simulink subsystem "rss_ShuntMeasurementCircuit"  (R2022b)
settings: Solver=VariableStepAuto  StartTime=0.0  StopTime=10.0  RelTol=1e-3
undefined symbols (not defined in the file): cstShntFiltRstn, cstShntRstn
libraries: fl_lib x10, nesl_utility x1
settings Model: Creator=CAV2OFO  LastModifiedBy=CAV2OFO

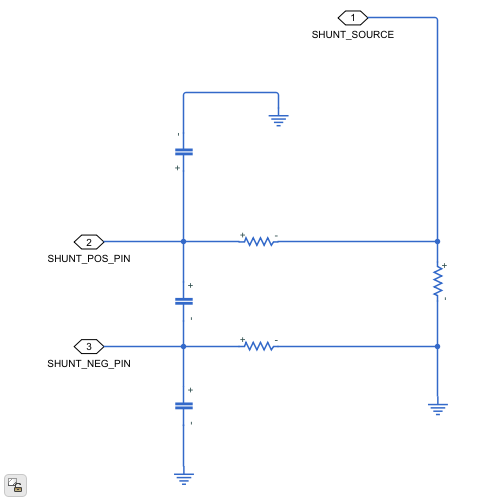
[thumbnail: Simulink's stored preview of the top-level diagram]
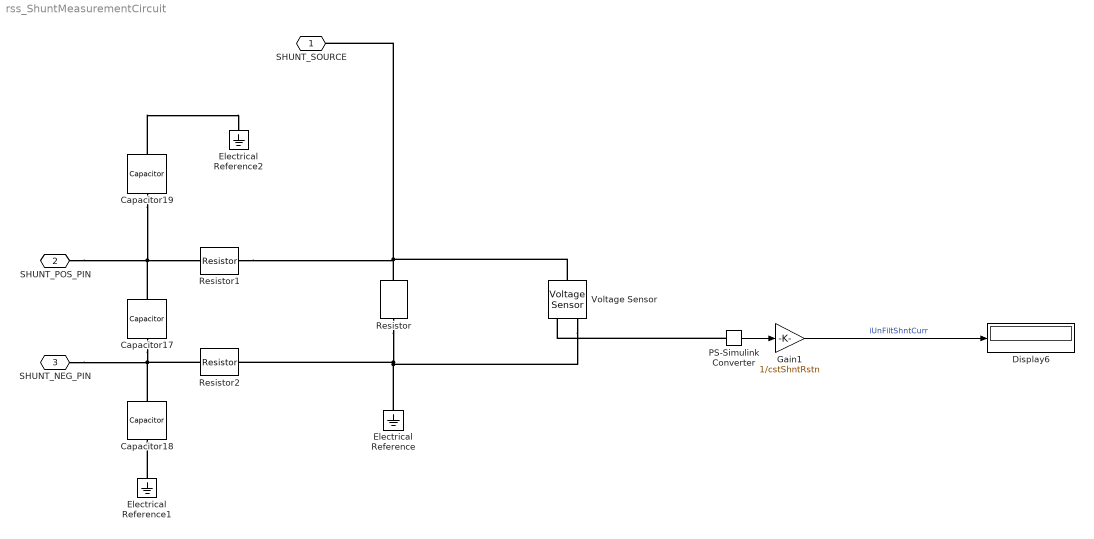
== system rss_ShuntMeasurementCircuit ==
  Capacitor17 : fl_lib/Electrical/Electrical Elements/Capacitor  c=cstShntCpct F  r=cstShntCpcrRstn Ohm  g=0 1/Ohm  i_specify=off  i_priority=None  i=0 A  i_nominal_specify=off  i_nominal_unit=A  i_nominal_value=1  v_specify=off  v_priority=None  v=0 V  v_nominal_specify=off  v_nominal_unit=V  v_nominal_value=1  vc_specify=off  vc_priority=High  vc=0 V  vc_nominal_specify=off  vc_nominal_unit=V  vc_nominal_value=1
  Capacitor18 : fl_lib/Electrical/Electrical Elements/Capacitor  c=cstShntGrndCpct F  r=cstShntGrndCpcrRstn Ohm  g=0 1/Ohm  i_specify=off  i_priority=None  i=0 A  i_nominal_specify=off  i_nominal_unit=A  i_nominal_value=1  v_specify=off  v_priority=None  v=0 V  v_nominal_specify=off  v_nominal_unit=V  v_nominal_value=1  vc_specify=off  vc_priority=High  vc=0 V  vc_nominal_specify=off  vc_nominal_unit=V  vc_nominal_value=1
  Capacitor19 : fl_lib/Electrical/Electrical Elements/Capacitor  c=cstShntGrndCpct F  r=cstShntGrndCpcrRstn Ohm  g=0 1/Ohm  i_specify=off  i_priority=None  i=0 A  i_nominal_specify=off  i_nominal_unit=A  i_nominal_value=1  v_specify=off  v_priority=None  v=0 V  v_nominal_specify=off  v_nominal_unit=V  v_nominal_value=1  vc_specify=off  vc_priority=High  vc=0 V  vc_nominal_specify=off  vc_nominal_unit=V  vc_nominal_value=1
  Display6 : Display
  Electrical Reference : fl_lib/Electrical/Electrical Elements/Electrical Reference
  Electrical Reference1 : fl_lib/Electrical/Electrical Elements/Electrical Reference
  Electrical Reference2 : fl_lib/Electrical/Electrical Elements/Electrical Reference
  Gain1 : Gain  Gain=1/cstShntRstn
  PS-Simulink Converter : nesl_utility/PS-Simulink Converter  PhysicalDomain=network_engine_domain  SubClassName=ps_output  LeftPortType=input  RightPortType=output  PseudoPeriodic=off  Frequencies=[]  VectorFormat=inherit  Unit=inherit  AffineConversion=off
  Resistor : fl_lib/Electrical/Electrical Elements/Resistor  R=cstShntRstn Ohm  i_specify=off  i_priority=None  i=0 A  i_nominal_specify=off  i_nominal_unit=A  i_nominal_value=1  v_specify=off  v_priority=None  v=0 V  v_nominal_specify=off  v_nominal_unit=V  v_nominal_value=1
  Resistor1 : fl_lib/Electrical/Electrical Elements/Resistor  R=cstShntFiltRstn Ohm  i_specify=off  i_priority=None  i=0 A  i_nominal_specify=off  i_nominal_unit=A  i_nominal_value=1  v_specify=off  v_priority=None  v=0 V  v_nominal_specify=off  v_nominal_unit=V  v_nominal_value=1
  Resistor2 : fl_lib/Electrical/Electrical Elements/Resistor  R=cstShntFiltRstn Ohm  i_specify=off  i_priority=None  i=0 A  i_nominal_specify=off  i_nominal_unit=A  i_nominal_value=1  v_specify=off  v_priority=None  v=0 V  v_nominal_specify=off  v_nominal_unit=V  v_nominal_value=1
  Voltage Sensor : fl_lib/Electrical/Electrical Sensors/Voltage Sensor
  SHUNT_SOURCE : PMIOPort  Side=Left
  SHUNT_POS_PIN : PMIOPort  Port=2  Side=Right
  SHUNT_NEG_PIN : PMIOPort  Port=3  Side=Right
  wires:
  PS-Simulink Converter/1 -> Gain1/1
  Gain1/1 -> Display6/1  "iUnFiltShntCurr"
  connections:
  Voltage Sensor/RConn2 -- Electrical Reference/LConn1 -- Resistor2/RConn1 -- Resistor/RConn1
  Voltage Sensor/LConn1 -- SHUNT_SOURCE/RConn1 -- Resistor1/RConn1 -- Resistor/LConn1
  Capacitor19/LConn1 -- Capacitor17/LConn1 -- SHUNT_POS_PIN/RConn1 -- Resistor1/LConn1
  Capacitor18/LConn1 -- Capacitor17/RConn1 -- SHUNT_NEG_PIN/RConn1 -- Resistor2/LConn1
  Electrical Reference1/LConn1 -- Capacitor18/RConn1
  Capacitor19/RConn1 -- Electrical Reference2/LConn1
  PS-Simulink Converter/LConn1 -- Voltage Sensor/RConn1
